simulink library "upChangeDetector"  (R2023b)
settings: Solver=VariableStepAuto  StartTime=0.0  StopTime=10.0  RelTol=1e-3
settings Model: Creator=muralikarnam  LastModifiedBy=User
settings SolverCC: AlgebraicLoopSolver=TrustRegion
settings DataIOCC: ReturnWorkspaceOutputs=off
settings DebuggingCC: UnconnectedInputMsg=warning  UnconnectedOutputMsg=warning  UnconnectedLineMsg=warning  ArithmeticOperatorsInVariantConditions=warning
settings ModelReferenceCC: EnableRefExpFcnMdlSchedulingChecks=on
settings SFSimCC: CustomCodeUndefinedFunction=UseInterfaceOnly

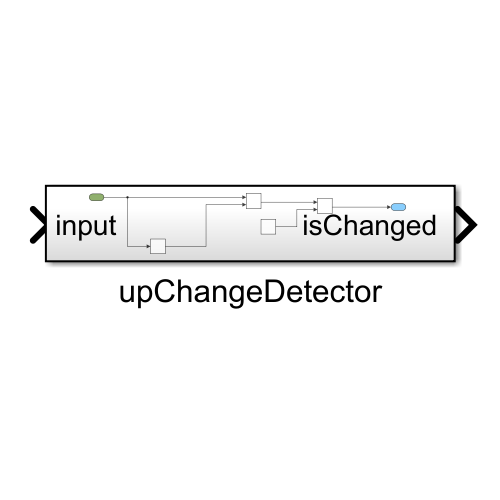
[thumbnail: Simulink's stored preview of the top-level diagram]
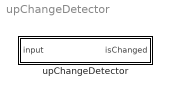
== system upChangeDetector ==
  upChangeDetector : Subsystem

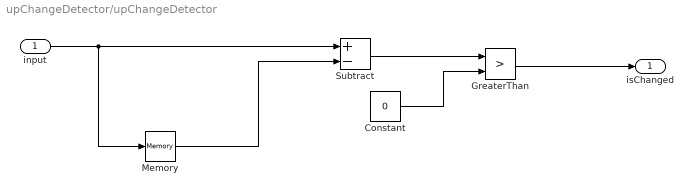
== system upChangeDetector/upChangeDetector ==
  input : Inport  PortDimensions=1
  Constant : Constant  Value=0
  GreaterThan : RelationalOperator  Operator=>  OutDataTypeStr=boolean  RndMeth=Simplest  InputSameDT=off
  Memory : Memory
  Subtract : Sum  Inputs=+-
  "isChanged " : Outport  OutDataTypeStr=boolean  PortDimensions=1  VectorParamsAs1DForOutWhenUnconnected=off
  wires:
  input/1 -> Memory/1, Subtract/1
  Memory/1 -> Subtract/2
  Subtract/1 -> GreaterThan/1
  Constant/1 -> GreaterThan/2
  GreaterThan/1 -> "isChanged "/1
